simulink model "BatteryModelChargingDischarging_1"  (R2025a)
settings: Solver=VariableStepAuto  StartTime=0.0  StopTime=0.1  RelTol=1e-3
undefined symbols (not defined in the file): C1, Np, Ns, Q, R0, R1
libraries: simulink x2, simulink_extras x1
settings Model: Creator=khan1  LastModifiedBy=arise
settings SolverCC: AlgebraicLoopSolver=TrustRegion
settings DataIOCC: ReturnWorkspaceOutputs=off
settings DebuggingCC: UnconnectedInputMsg=warning  UnconnectedOutputMsg=warning  UnconnectedLineMsg=warning  ArithmeticOperatorsInVariantConditions=warning
settings ModelReferenceCC: EnableRefExpFcnMdlSchedulingChecks=on
settings SFSimCC: SimUseLocalCustomCode=off  CustomCodeUndefinedFunction=UseInterfaceOnly
settings RTWCC: RTWUseLocalCustomCode=off  GPUComputeCapability=3.5

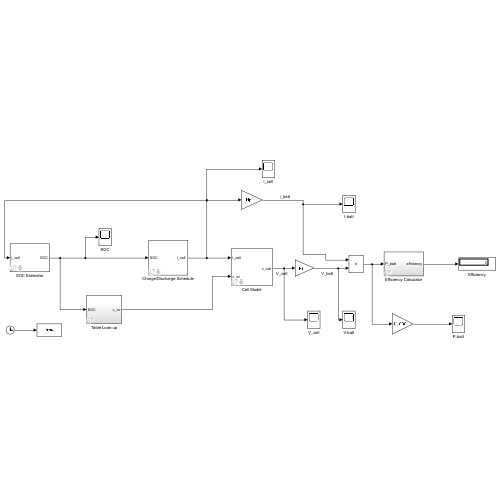
[thumbnail: Simulink's stored preview of the top-level diagram]
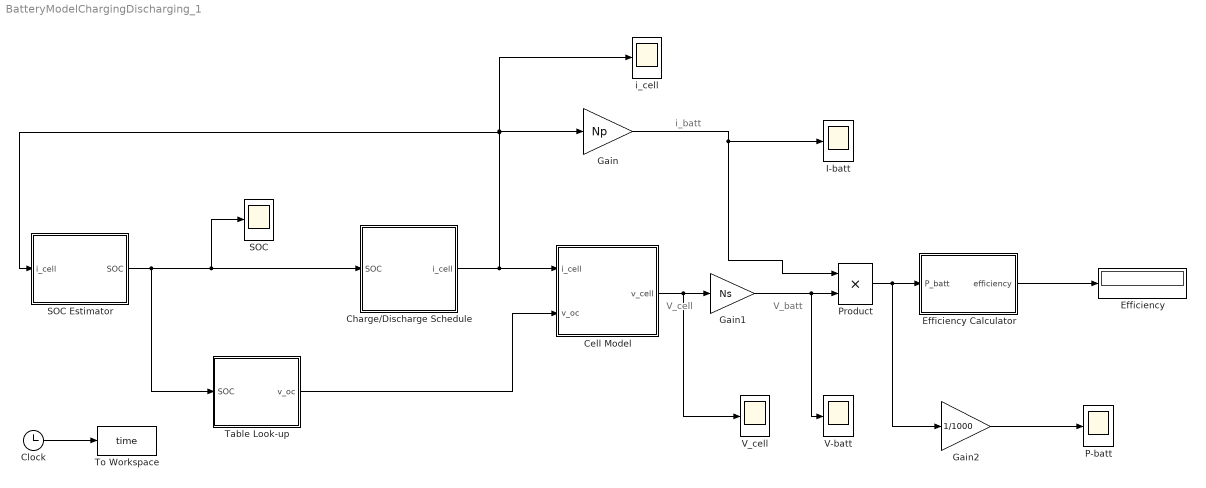
== system BatteryModelChargingDischarging_1 ==
  note: i_batt
  note: V_batt
  note: V_cell
  Cell Model : Subsystem  AncestorBlock=Project4_lib_2015b/Cell Model  mask{R0=R0, R1=R1, C1=C1}
  Charge/Discharge Schedule : Subsystem  AncestorBlock=Project4_lib_2015b/Charge//Discharge Schedule  mask{c_rate_charge=2, c_rate_discharge=2, SOC_max=.95, SOC_min=.2}
  Clock : Clock
  Efficiency : Display
  Efficiency Calculator : Subsystem  AncestorBlock=Project4_lib_2015b/Efficiency Calculator
  Gain : Gain  Gain=Np
  Gain1 : Gain  Gain=Ns
  Gain2 : Gain  Gain=1/1000
  I-batt : Scope
      settings: ActiveDisplayYMinimum=-72  ActiveDisplayYMaximum=-52  DataLoggingVariableName=ibatt  DataLoggingSaveFormat=Structure
  P-batt : Scope
      settings: ActiveDisplayYMinimum=-20.674391516352529  ActiveDisplayYMaximum=-20.673156498183051  DataLoggingVariableName=pbatt  DataLoggingSaveFormat=Structure
  Product : Product
  SOC : Scope
      settings: ActiveDisplayYMinimum=0.19999305555555552  ActiveDisplayYMaximum=0.2000625000000005  DataLoggingVariableName=soc  DataLoggingSaveFormat=Structure
  SOC Estimator : Subsystem  AncestorBlock=Project4_lib_2015b/SOC Estimator  mask{SOC_init=.2}
  Table Look-up : Subsystem  AncestorBlock=Project4_lib_2015b/Table Look-up
  To Workspace : ToWorkspace  VariableName=time  SaveFormat=Timeseries  SampleTime=-1
  V-batt : Scope
      settings: ActiveDisplayYMinimum=333.43822799667305  ActiveDisplayYMaximum=333.4559480299427  DataLoggingVariableName=vbatt  DataLoggingSaveFormat=Structure
  V_cell : Scope
      settings: ActiveDisplayYMinimum=4.167975100440132  ActiveDisplayYMaximum=4.1682240960388155  DataLoggingSaveFormat=Structure
  i_cell : Scope
      settings: ActiveDisplayYMinimum=-72  ActiveDisplayYMaximum=-52
  wires:
  SOC Estimator/1(SOC) -> Table Look-up/1(SOC), SOC/1, Charge/Discharge Schedule/1(SOC)
  Charge/Discharge Schedule/1("i_cell ") -> i_cell/1, Gain/1, SOC Estimator/1(i_cell), Cell Model/1(i_cell)
  Cell Model/1(v_cell) -> V_cell/1, Gain1/1
  Gain/1 -> I-batt/1, Product/1
  Table Look-up/1(v_oc) -> Cell Model/2("v_oc ")
  Product/1 -> Gain2/1, Efficiency Calculator/1(P_batt)
  Efficiency Calculator/1(efficiency) -> Efficiency/1
  Gain1/1 -> V-batt/1, Product/2
  Clock/1 -> To Workspace/1
  Gain2/1 -> P-batt/1

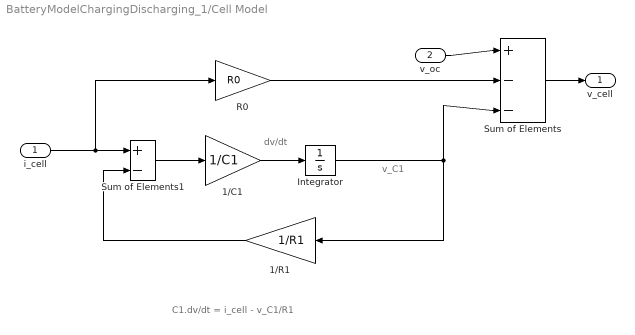
== system BatteryModelChargingDischarging_1/Cell Model ==
  note: C1.dv/dt = i_cell - v_C1/R1
  note: dv/dt
  note: v_C1
  i_cell : Inport
  "v_oc " : Inport  Port=2
  1/C1 : Gain  Gain=1/C1
  1/R1 : Gain  Gain=1/R1
  Integrator : Integrator
  R0 : Gain  Gain=R0
  Sum of Elements : Sum  Inputs=+--
  Sum of Elements1 : Sum  Inputs=+-
  v_cell : Outport  VectorParamsAs1DForOutWhenUnconnected=off
  wires:
  Integrator/1 -> Sum of Elements/3, 1/R1/1
  1/R1/1 -> Sum of Elements1/2
  Sum of Elements/1 -> v_cell/1
  1/C1/1 -> Integrator/1
  Sum of Elements1/1 -> 1/C1/1
  R0/1 -> Sum of Elements/2
  "v_oc "/1 -> Sum of Elements/1
  i_cell/1 -> Sum of Elements1/1, R0/1

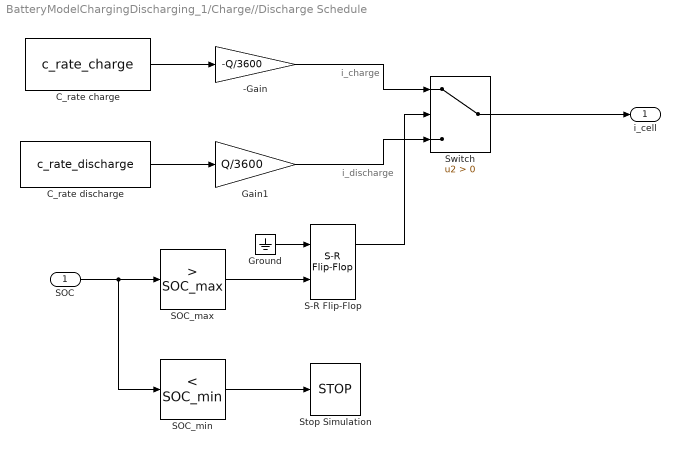
== system BatteryModelChargingDischarging_1/Charge//Discharge Schedule ==
  note: i_charge
  note: i_discharge
  SOC : Inport
  -Gain : Gain  Gain=-Q/3600
  C_rate charge : Constant  Value=c_rate_charge
  C_rate discharge : Constant  Value=c_rate_discharge
  Gain1 : Gain  Gain=Q/3600
  Ground : Ground
  S-R Flip-Flop : simulink_extras/Flip Flops/S-R Flip-Flop  initial_condition=1
  "SOC_max " : simulink/Logic and Bit Operations/Compare To Constant  relop=>  const=SOC_max  OutDataTypeStr=boolean
  SOC_min : simulink/Logic and Bit Operations/Compare To Constant  relop=<  const=SOC_min  OutDataTypeStr=boolean
  Stop Simulation : Stop
  Switch : Switch  Criteria=u2 > Threshold  SaturateOnIntegerOverflow=off  InputSameDT=off
  "i_cell " : Outport  VectorParamsAs1DForOutWhenUnconnected=off
  wires:
  Ground/1 -> S-R Flip-Flop/1
  Switch/1 -> "i_cell "/1
  SOC_min/1 -> Stop Simulation/1
  SOC/1 -> "SOC_max "/1, SOC_min/1
  "SOC_max "/1 -> S-R Flip-Flop/2
  S-R Flip-Flop/1 -> Switch/2
  Gain1/1 -> Switch/3
  -Gain/1 -> Switch/1
  C_rate discharge/1 -> Gain1/1
  C_rate charge/1 -> -Gain/1

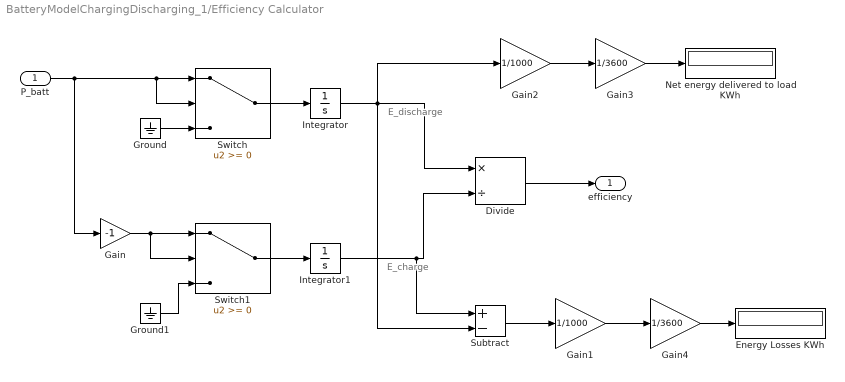
== system BatteryModelChargingDischarging_1/Efficiency Calculator ==
  note: E_discharge
  note: E_charge
  P_batt : Inport
  Divide : Product  Inputs=*/
  Energy Losses KWh : Display
  Gain : Gain  Gain=-1
  Gain1 : Gain  Gain=1/1000
  Gain2 : Gain  Gain=1/1000
  Gain3 : Gain  Gain=1/3600
  Gain4 : Gain  Gain=1/3600
  Ground : Ground
  Ground1 : Ground
  Integrator : Integrator
  Integrator1 : Integrator
  Net energy delivered to load KWh : Display
  Subtract : Sum  Inputs=+-
  Switch : Switch  SaturateOnIntegerOverflow=off  InputSameDT=off
  Switch1 : Switch  SaturateOnIntegerOverflow=off  InputSameDT=off
  efficiency : Outport  VectorParamsAs1DForOutWhenUnconnected=off
  wires:
  Divide/1 -> efficiency/1
  Integrator1/1 -> Subtract/1, Divide/2
  Integrator/1 -> Divide/1, Gain2/1, Subtract/2
  Switch1/1 -> Integrator1/1
  Switch/1 -> Integrator/1
  Ground1/1 -> Switch1/3
  Gain/1 -> Switch1/1, Switch1/2
  Ground/1 -> Switch/3
  P_batt/1 -> Switch/1, Switch/2, Gain/1
  Gain3/1 -> Net energy delivered to load KWh/1
  Gain2/1 -> Gain3/1
  Gain1/1 -> Gain4/1
  Gain4/1 -> Energy Losses KWh/1
  Subtract/1 -> Gain1/1

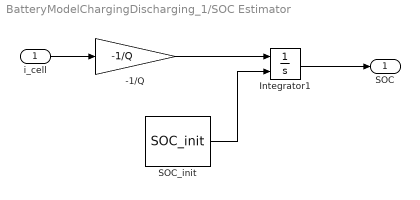
== system BatteryModelChargingDischarging_1/SOC Estimator ==
  i_cell : Inport
  -1/Q : Gain  Gain=-1/Q
  Integrator1 : Integrator  InitialConditionSource=external
  SOC_init : Constant  Value=SOC_init
  SOC : Outport  VectorParamsAs1DForOutWhenUnconnected=off
  wires:
  SOC_init/1 -> Integrator1/2
  Integrator1/1 -> SOC/1
  -1/Q/1 -> Integrator1/1
  i_cell/1 -> -1/Q/1

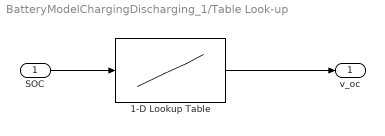
== system BatteryModelChargingDischarging_1/Table Look-up ==
  SOC : Inport
  1-D Lookup Table : Lookup_n-D  NumberOfTableDimensions=1  BreakpointsForDimension1=[0 0.1 0.25 0.5 0.75 0.9 1]  Table="[ 3.51  3.57  3.63  3.71  3.93  4.08  4.19]"  RndMeth=Simplest
  v_oc : Outport  VectorParamsAs1DForOutWhenUnconnected=off
  wires:
  1-D Lookup Table/1 -> v_oc/1
  SOC/1 -> 1-D Lookup Table/1
